simulink model "fleet_test"  (R2025b)
settings: Solver=VariableStepAuto  StartTime=0.0  StopTime=200  RelTol=1e-3
settings Model: Creator=sanborkl  LastModifiedBy=admin

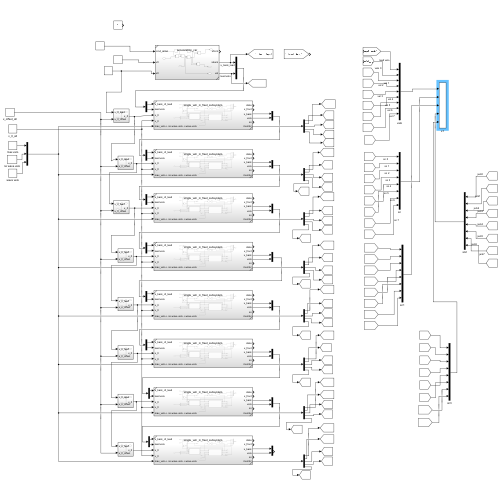
[thumbnail: Simulink's stored preview of the top-level diagram]
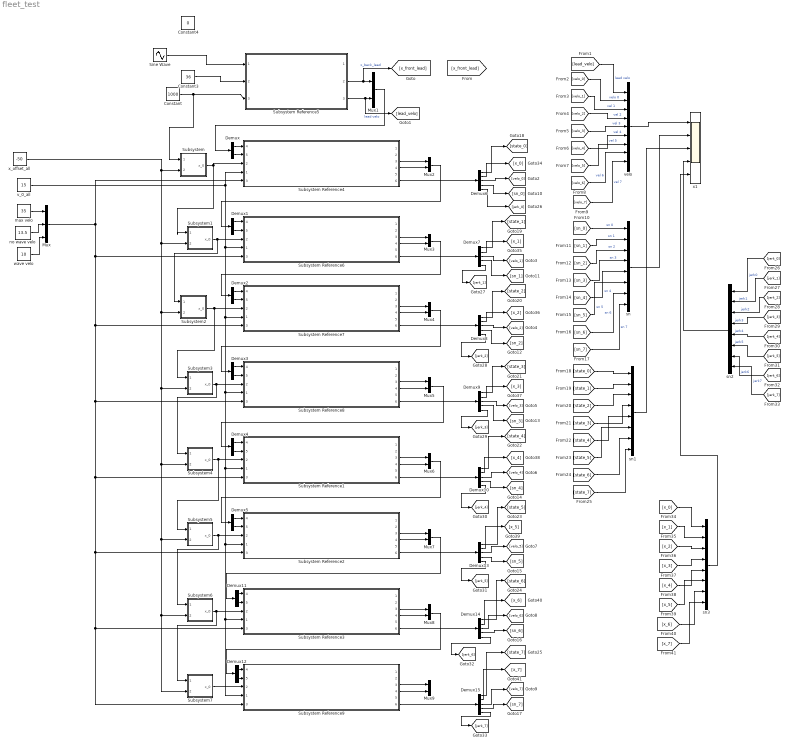
== system fleet_test ==
  Constant : Constant  Value=1000
  Constant3 : Constant  Value=36
  Constant4 : Constant  Value=0
  Demux{,1..5,11..12} (8 alike) : Demux  Outputs=2
  Demux{6..10,13..15} (8 alike) : Demux  Outputs=5
  Mux : Mux  Inputs=3
  Mux{1..9} (9 alike) : Mux  Inputs=2
  Sine Wave : Sin  Amplitude=2  SampleTime=0
  Subsystem : Subsystem
  Subsystem Reference{1..4,6..9} (8 alike) : Subsystem  ReferencedSubsystem=single_veh_in_fleet_subsystem
      settings: PortSchema="{\"entries\":[{\"content\":{\"sides\":[{\"content\":{\"connectorIds\":[\"In4\",\"In5\",\"In2\",\"In1\",\"In3\"]},\"type\":\"ConnectorPlacement.EquallySpacedRectSide\",\"uuid\":\"b0c0edea-aecf-47b9-8232-de471d45dacc\"},{\"content\":{\"connectorIds\":[\"Out1\",\"Out2\",\"Out3\",\"Out4\",\"Out5\",\"Out6\"],\"side\":\"RIGHT\"},\"type\":\"ConnectorPlacement.EquallySpacedRectSide\",\"uuid\":\"e7164750-1794-4fbe-9c7b-d29abe843a07\"},{\"content\":{\"side\":\"TOP\"},\"type\":\"ConnectorPlacement.EquallySpacedRectSide\",\"uuid\":\"eb44f96e-f8ec-45f8-beb0-67b14a0c8794\"}]},\"type\":\"ConnectorPlacement.EquallySpacedConnector\",\"uuid\":\"4d437575-c71d-4bca-a6ac-bb17cb48b595\"}],\"packageUris\":[\"http://schema.mathworks.com/mf0/Connector/R2020b\"],\"version\":\"1.0\"}"
  Subsystem Reference5 : Subsystem  ReferencedSubsystem=acceleration_car
  Subsystem1 : Subsystem
  Subsystem2 : Subsystem
  Subsystem3 : Subsystem
  Subsystem4 : Subsystem
  Subsystem5 : Subsystem
  Subsystem6 : Subsystem
  Subsystem7 : Subsystem
  max velo : Constant  Value=35
  no wave velo : Constant  Value=13.5
  sn{,1..3} (4 alike) : Mux  Inputs=8
  v_0_all : Constant  Value=15
  velo : Mux  Inputs=9
  wave velo : Constant  Value=10
  x1 : Scope  NumInputPorts=5
      settings: ActiveDisplayYMinimum=11.875771193485413  ActiveDisplayYMaximum=43.1180592586313  DataLoggingVariableName=ScopeData7
  x_offset_all : Constant  Value=-50
  wires:
  Constant3/1 -> Subsystem Reference5/2
  x_offset_all/1 -> Subsystem7/2(x_0_offset), Subsystem6/2(x_0_offset), Subsystem5/2(x_0_offset), Subsystem4/2(x_0_offset), Subsystem3/2(x_0_offset), Subsystem2/2(x_0_offset), Subsystem1/2(x_0_offset), Subsystem/2(x_0_offset)
  max velo/1 -> Mux/1
  no wave velo/1 -> Mux/2
  wave velo/1 -> Mux/3
  Mux/1 -> Subsystem Reference6/3, Subsystem Reference9/3, Subsystem Reference3/3, Subsystem Reference2/3, Subsystem Reference1/3, Subsystem Reference8/3, Subsystem Reference7/3, Subsystem Reference4/3
  Subsystem/1(x_0) -> Subsystem1/1(x_0_lead), Subsystem Reference4/2
  v_0_all/1 -> Subsystem Reference6/1, Subsystem Reference2/1, Subsystem Reference9/1, Subsystem Reference3/1, Subsystem Reference1/1, Subsystem Reference8/1, Subsystem Reference7/1, Subsystem Reference4/1
  Subsystem Reference5/2 -> [x_front_lead], Mux1/1  "x_back_lead"
  Subsystem Reference5/3 -> [lead_velo], Mux1/2  "lead velo"
  Demux/1 -> Subsystem Reference4/4
  Demux/2 -> Subsystem Reference4/5
  Mux1/1 -> Demux/1
  Subsystem Reference4/3 -> Mux2/1
  Subsystem Reference4/4 -> Mux2/2
  Subsystem Reference6/4 -> Mux3/2
  Subsystem Reference6/3 -> Mux3/1
  Demux1/2 -> Subsystem Reference6/5
  Demux1/1 -> Subsystem Reference6/4
  Mux2/1 -> Demux1/1
  Subsystem1/1(x_0) -> Subsystem2/1(x_0_lead), Subsystem Reference6/2
  Subsystem Reference7/4 -> Mux4/2
  Subsystem Reference7/3 -> Mux4/1
  Demux2/2 -> Subsystem Reference7/5
  Demux2/1 -> Subsystem Reference7/4
  Subsystem2/1(x_0) -> Subsystem Reference7/2, Subsystem3/1(x_0_lead)
  Sine Wave/1 -> Subsystem Reference5/1
  [lead_velo] -> velo/1  "lead velo"
  [velo_0] -> velo/2  "velo 0"
  [velo_1] -> velo/3  "vel 1"
  [velo_2] -> velo/4  "vel 2"
  [velo_3] -> velo/5  "vel 3"
  [velo_4] -> velo/6  "vel 4"
  [velo_5] -> velo/7  "vel 5"
  [velo_6] -> velo/8  "vel 6"
  [velo_7] -> velo/9  "vel 7"
  velo/1 -> x1/1
  [sn_0] -> sn/1  "sn 0"
  [sn_1] -> sn/2  "sn 1"
  [sn_2] -> sn/3  "sn 2"
  [sn_3] -> sn/4  "sn 3"
  [sn_4] -> sn/5  "sn 4"
  [sn_5] -> sn/6  "sn 5"
  [sn_6] -> sn/7  "sn 6"
  [sn_7] -> sn/8  "sn 7"
  sn/1 -> x1/2
  [state_0] -> sn1/1
  [state_1] -> sn1/2
  [state_2] -> sn1/3
  [state_3] -> sn1/4
  [state_4] -> sn1/5
  [state_5] -> sn1/6
  [state_6] -> sn1/7
  [state_7] -> sn1/8
  Mux4/1 -> Demux3/1
  Mux3/1 -> Demux2/1
  Subsystem3/1(x_0) -> Subsystem4/1(x_0_lead), Subsystem Reference8/2
  Demux3/1 -> Subsystem Reference8/4
  Demux3/2 -> Subsystem Reference8/5
  Subsystem Reference8/3 -> Mux5/1
  Demux4/1 -> Subsystem Reference1/4
  Demux4/2 -> Subsystem Reference1/5
  Subsystem4/1(x_0) -> Subsystem5/1(x_0_lead), Subsystem Reference1/2
  Mux5/1 -> Demux4/1
  Demux5/2 -> Subsystem Reference2/5
  Demux5/1 -> Subsystem Reference2/4
  Subsystem Reference1/3 -> Mux6/1
  Subsystem Reference1/4 -> Mux6/2
  Mux6/1 -> Demux5/1
  Subsystem Reference8/4 -> Mux5/2
  Subsystem Reference4/6 -> Demux6/1
  Demux6/1 -> [state_0]
  Demux6/3 -> [velo_0]
  Demux6/4 -> [sn_0]
  Subsystem Reference6/6 -> Demux7/1
  Demux7/1 -> [state_1]
  Demux7/3 -> [velo_1]
  Demux7/4 -> [sn_1]
  Subsystem Reference7/6 -> Demux8/1
  Demux8/1 -> [state_2]
  Demux8/3 -> [velo_2]
  Demux8/4 -> [sn_2]
  Subsystem Reference8/6 -> Demux9/1
  Demux9/1 -> [state_3]
  Demux9/3 -> [velo_3]
  Demux9/4 -> [sn_3]
  Subsystem Reference1/6 -> Demux10/1
  Demux10/1 -> [state_4]
  Demux10/3 -> [velo_4]
  Demux10/4 -> [sn_4]
  Subsystem Reference2/3 -> Mux7/1
  Subsystem Reference2/4 -> Mux7/2
  Subsystem Reference3/4 -> Mux8/2
  Subsystem Reference3/3 -> Mux8/1
  Mux7/1 -> Demux11/1
  Demux11/1 -> Subsystem Reference3/4
  Demux11/2 -> Subsystem Reference3/5
  Subsystem Reference9/3 -> Mux9/1
  Subsystem Reference9/4 -> Mux9/2
  Mux8/1 -> Demux12/1
  Demux12/1 -> Subsystem Reference9/4
  Demux12/2 -> Subsystem Reference9/5
  Subsystem Reference2/6 -> Demux13/1
  Demux13/1 -> [state_5]
  Demux13/3 -> [velo_5]
  Demux13/4 -> [sn_5]
  Subsystem Reference3/6 -> Demux14/1
  Demux14/1 -> [state_6]
  Demux14/3 -> [velo_6]
  Demux14/4 -> [sn_6]
  Demux15/4 -> [sn_7]
  Demux15/3 -> [velo_7]
  Demux15/1 -> [state_7]
  Subsystem Reference9/6 -> Demux15/1
  Subsystem5/1(x_0) -> Subsystem6/1(x_0_lead), Subsystem Reference2/2
  Subsystem6/1(x_0) -> Subsystem7/1(x_0_lead), Subsystem Reference3/2
  Subsystem7/1(x_0) -> Subsystem Reference9/2
  Constant/1 -> Subsystem/1(x_0_lead), Subsystem Reference5/3
  Demux6/5 -> [jerk_0]
  Demux7/5 -> [jerk_1]
  Demux8/5 -> [jerk_2]
  Demux9/5 -> [jerk_3]
  Demux10/5 -> [jerk_4]
  Demux13/5 -> [jerk_5]
  Demux14/5 -> [jerk_6]
  Demux15/5 -> [jerk_7]
  [jerk_0] -> sn2/1  "jerk0"
  [jerk_1] -> sn2/2  "jerk1"
  [jerk_2] -> sn2/3  "jerk2"
  [jerk_3] -> sn2/4  "jerk3"
  [jerk_4] -> sn2/5  "jerk4"
  [jerk_5] -> sn2/6  "jerk5"
  [jerk_6] -> sn2/7  "jerk6"
  [jerk_7] -> sn2/8  "jerk7"
  sn2/1 -> x1/4
  Demux6/2 -> [x_0]
  Demux7/2 -> [x_1]
  Demux8/2 -> [x_2]
  Demux9/2 -> [x_3]
  Demux10/2 -> [x_4]
  Demux13/2 -> [x_5]
  Demux14/2 -> [x_6]
  Demux15/2 -> [x_7]
  [x_0] -> sn3/1
  [x_1] -> sn3/2
  [x_2] -> sn3/3
  [x_3] -> sn3/4
  [x_4] -> sn3/5
  [x_5] -> sn3/6
  [x_6] -> sn3/7
  [x_7] -> sn3/8
  sn3/1 -> x1/5
  sn1/1 -> x1/3

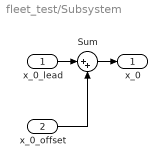
== system fleet_test/Subsystem ==
  x_0_lead : Inport
  x_0_offset : Inport  Port=2
  Sum : Sum  Inputs=|++
  x_0 : Outport
  wires:
  x_0_lead/1 -> Sum/1
  Sum/1 -> x_0/1
  x_0_offset/1 -> Sum/2

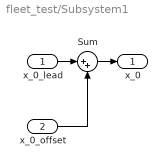
== system fleet_test/Subsystem1 ==
  x_0_lead : Inport
  x_0_offset : Inport  Port=2
  Sum : Sum  Inputs=|++
  x_0 : Outport
  wires:
  x_0_offset/1 -> Sum/2
  Sum/1 -> x_0/1
  x_0_lead/1 -> Sum/1

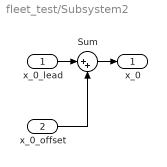
== system fleet_test/Subsystem2 ==
  x_0_lead : Inport
  x_0_offset : Inport  Port=2
  Sum : Sum  Inputs=|++
  x_0 : Outport
  wires:
  x_0_offset/1 -> Sum/2
  Sum/1 -> x_0/1
  x_0_lead/1 -> Sum/1

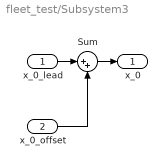
== system fleet_test/Subsystem3 ==
  x_0_lead : Inport
  x_0_offset : Inport  Port=2
  Sum : Sum  Inputs=|++
  x_0 : Outport
  wires:
  x_0_lead/1 -> Sum/1
  Sum/1 -> x_0/1
  x_0_offset/1 -> Sum/2

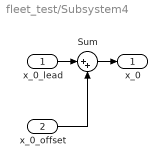
== system fleet_test/Subsystem4 ==
  x_0_lead : Inport
  x_0_offset : Inport  Port=2
  Sum : Sum  Inputs=|++
  x_0 : Outport
  wires:
  x_0_offset/1 -> Sum/2
  Sum/1 -> x_0/1
  x_0_lead/1 -> Sum/1

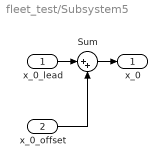
== system fleet_test/Subsystem5 ==
  x_0_lead : Inport
  x_0_offset : Inport  Port=2
  Sum : Sum  Inputs=|++
  x_0 : Outport
  wires:
  x_0_lead/1 -> Sum/1
  Sum/1 -> x_0/1
  x_0_offset/1 -> Sum/2

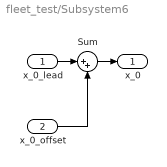
== system fleet_test/Subsystem6 ==
  x_0_lead : Inport
  x_0_offset : Inport  Port=2
  Sum : Sum  Inputs=|++
  x_0 : Outport
  wires:
  x_0_offset/1 -> Sum/2
  Sum/1 -> x_0/1
  x_0_lead/1 -> Sum/1

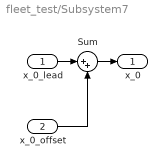
== system fleet_test/Subsystem7 ==
  x_0_lead : Inport
  x_0_offset : Inport  Port=2
  Sum : Sum  Inputs=|++
  x_0 : Outport
  wires:
  x_0_lead/1 -> Sum/1
  Sum/1 -> x_0/1
  x_0_offset/1 -> Sum/2
